simulink model "Fault_analysis_of_3phase"  (R2020a)
settings: Solver=VariableStepAuto  StartTime=0.0  StopTime=0.6  RelTol=1e-3
libraries: powerlib x6, simulink_extras x3
settings Model: Creator=Reaga  LastModifiedBy=Reaga
settings DebuggingCC: UnconnectedInputMsg=none  UnconnectedOutputMsg=none  UnconnectedLineMsg=none
settings ModelReferenceCC: EnableRefExpFcnMdlSchedulingChecks=off
settings RTWCC: Description=Generic Real-Time Target
settings ConfigComp: CovBoundaryAbsTol=1.0e-5

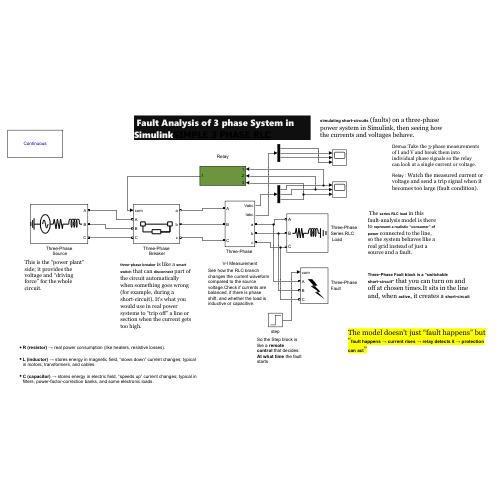
[thumbnail: Simulink's stored preview of the top-level diagram]
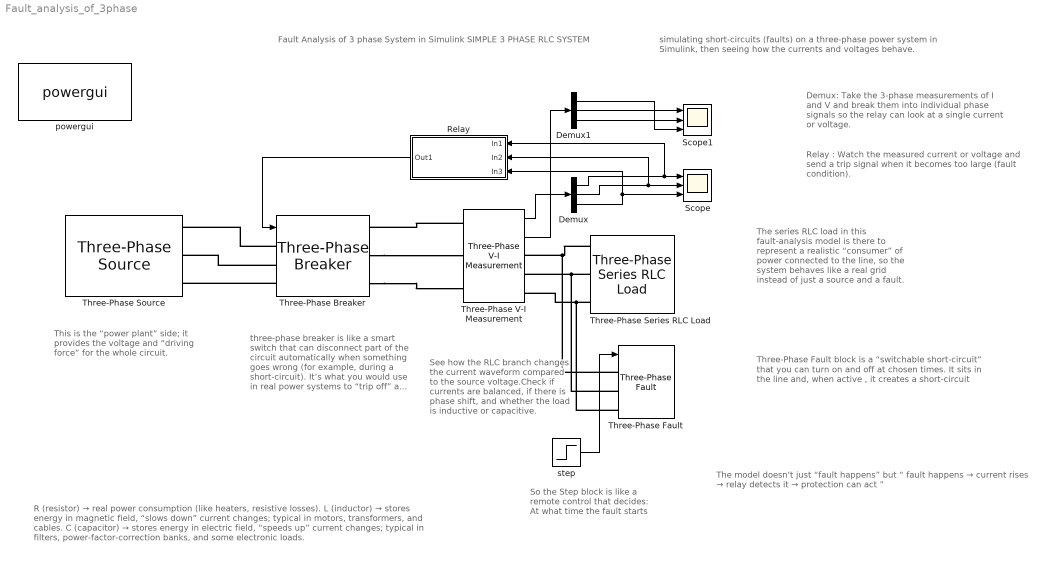
== system Fault_analysis_of_3phase ==
  note: The model doesn't just “fault happens” but “ fault happens → current rises → relay detects it → protection can act ”
  note: Relay : Watch the measured current or voltage and send a trip signal when it becomes too large (fault condition).
  note: Demux: Take the 3‑phase measurements of I and V and break them into individual phase signals so the relay can look at a single current or voltage.
  note: Three‑Phase Fault block is a “switchable short‑circuit” that you can turn on and off at chosen times. It sits in the line and, when active , it creates a short‑circuit
  note: So the Step block is like a remote control that decides:
      | At what time the fault starts
  note: The series RLC load in this fault‑analysis model is there to represent a realistic “consumer” of power connected to the line, so the system behaves like a real grid instead of just a source and a fault.
  note: three‑phase breaker is like a smart switch that can disconnect part of the circuit automatically when something goes wrong (for example, during a short‑circuit). It’s what you would use in real power systems to “trip off” a line or section when the current gets too high.
  note: simulating short‑circuits (faults) on a three‑phase power system in Simulink, then seeing how the currents and voltages behave.
  note: See how the RLC branch changes the current waveform compared to the source voltage.Check if currents are balanced, if there is phase shift, and whether the load is inductive or capacitive.
  note: R (resistor) → real power consumption (like heaters, resistive losses).
      | L (inductor) → stores energy in magnetic field, “slows down” current changes; typical in motors, transformers, and cables.
      | C (capacitor) → stores energy in electric field, “speeds up” current changes; typical in filters, power‑factor‑correction banks, and some electronic loads.
  note: This is the “power plant” side; it provides the voltage and “driving force” for the whole circuit.
  note: Fault Analysis of 3 phase System in Simulink SIMPLE 3 PHASE RLC SYSTEM
  Demux : Demux  Outputs=3
  Demux1 : Demux  Outputs=3
  "Relay " : Subsystem
  Scope : Scope  NumInputPorts=3
  Scope1 : Scope  NumInputPorts=3
  Three-Phase Breaker : powerlib/Elements/Three-Phase Breaker  InitialState=closed  SwitchA=on  SwitchB=on  SwitchC=on  SwitchTimes="[1/60  5/60]"  External=on  BreakerResistance=0.001  SnubberResistance=1e6  SnubberCapacitance=inf  Measurements=None
  Three-Phase Source : powerlib/Electrical Sources/Three-Phase Source  InternalConnection=Yg  VoltagePhases=off  Voltage=11e3  PhaseAngle=0  Voltage_phases=[25e3 25e3 25e3]/sqrt(3)  PhaseAngles_phases=[0 -120 +120]  Frequency=60  NonIdealSource=on  SpecifyImpedance=off  Resistance=1e-3  Inductance=1e-6  ShortCircuitLevel=100e6  BaseVoltage=11e3  XRratio=7  BusType=swing  Pref=10e3  Qref=0  Prefabc=[10e3, 10e3, 10e3]  Qrefabc=[0, 0, 0]  Qmin=-inf  Qmax=inf
  Three-Phase Series RLC Load : powerlib/Elements/Three-Phase Series RLC Load  LConnTagsString=A|B|C  Configuration=Y (grounded)  NominalVoltage=11e3  Vabc=[1e3 1e3 1e3]  Vabcp=[1e3 1e3 1e3]  NominalFrequency=50  UnbalancedPower=off  ActivePower=200e6  InductivePower=100  CapacitivePower=0  Pabc=[10e3 9e3 11e3]  QLabc=[100 90 110]  QCabc=[100 90 110]  Pabcp=[10e3 9e3 11e3]  QLabcp=[100 90 110]  QCabcp=[100 90 110]  Measurements=None  LoadType=constant Z
  Three-Phase V-I Measurement : powerlib/Measurements/Three-Phase V-I Measurement  VoltageMeasurement=phase-to-phase  SetLabelV=off  LabelV=Vabc  Vpu=off  VpuLL=off  CurrentMeasurement=yes  SetLabelI=off  LabelI=Iabc  Ipu=off  Pbase=100e6  Vbase=500e3  OutputType=Complex  PhasorSimulation=off  PSBequivalent=0
  Three-Phase Fault : powerlib/Elements/Three-Phase Fault  InitialStates=[0 0 0]  FaultA=on  FaultB=on  FaultC=on  GroundFault=on  SwitchTimes="[1/60  5/60]"  External=on  SwitchStatus=NaN  FaultResistance=0.001  GroundResistance=0.01  SnubberResistance=1e6  SnubberCapacitance=inf  Measurements=None
  powergui : powerlib/powergui  Priority=1  SimulationMode=Continuous  SampleTime=50e-6  frequency=60  Iterations=50  frequencyindice=60  Pbase=100e6  ErrMax=1e-4  UnitsV=kV  UnitsW=MW  buscounter=0  FunctionMessages=off  echomessages=off  EnableUseOfTLC=off  CurrentSourceSwitches=off  DisableSnubberDevices=off  DisableRonSwitches=off  DisableVfSwitches=off  DisplayEquations=off  AutomaticDiscreteSolvers=off  SolverType=Tustin/Backward Euler (TBE)  Interpol=off  ExternalGateDelay=off  methode=off  Ts=100  x0status=blocks  SPID=on  SwTol=0  HookPort=off  NonlinearTolerance=1e-4  nMaxIteration=100  ContinueOnMaxIteration=off  RestoreLinks=warning  ResistiveCurrentMeasurement=off  Frange=[0:2:500]  Ylog=off  Xlog=on  ShowGrid=off  save=off  variable=ZData  structure=0  ZoomFFT=off  StartTime=0.0  cycles=1  DisplayStyle=1  fundamental=60  FreqAxis=off  MaxFrequency=1000  frequencyindicesteady=1  RmsSteady=1  display=off
  step : Step  Time=0.1  SampleTime=0
  wires:
  step/1 -> Three-Phase Fault/1
  "Relay "/1(Out1) -> Three-Phase Breaker/1
  Demux1/1 -> Scope1/3
  Demux1/2 -> Scope1/1
  Demux1/3 -> Scope1/2
  Demux/1 -> "Relay "/1(In1), Scope/1
  Demux/2 -> "Relay "/2(In2), Scope/2
  Demux/3 -> "Relay "/3(In3), Scope/3
  Three-Phase V-I Measurement/1 -> Demux/1
  Three-Phase V-I Measurement/2 -> Demux1/1
  connections:
  Three-Phase Breaker/LConn1 -- Three-Phase Source/RConn1
  Three-Phase Breaker/LConn2 -- Three-Phase Source/RConn2
  Three-Phase Breaker/LConn3 -- Three-Phase Source/RConn3
  Three-Phase Series RLC Load/LConn2 -- Three-Phase Fault/LConn2 -- Three-Phase V-I Measurement/RConn2
  Three-Phase Series RLC Load/LConn1 -- Three-Phase Fault/LConn1 -- Three-Phase V-I Measurement/RConn1
  Three-Phase Series RLC Load/LConn3 -- Three-Phase Fault/LConn3 -- Three-Phase V-I Measurement/RConn3
  Three-Phase V-I Measurement/LConn1 -- Three-Phase Breaker/RConn1
  Three-Phase Breaker/RConn2 -- Three-Phase V-I Measurement/LConn2
  Three-Phase Breaker/RConn3 -- Three-Phase V-I Measurement/LConn3

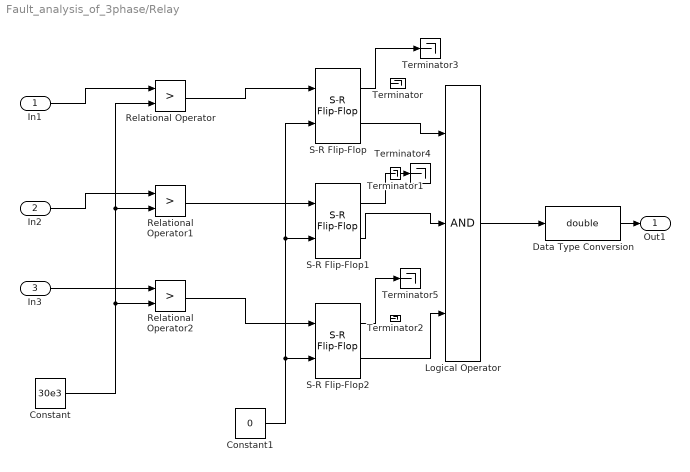
== system Fault_analysis_of_3phase/Relay  ==
  In1 : Inport
  In2 : Inport  Port=2
  In3 : Inport  Port=3
  Constant : Constant  Value=30e3
  Constant1 : Constant  Value=0  OutDataTypeStr=boolean
  Data Type Conversion : DataTypeConversion  OutDataTypeStr=double
  Logical Operator : Logic  Inputs=3  AllPortsSameDT=off  OutDataTypeStr=boolean
  Relational Operator : RelationalOperator  Operator=>  OutDataTypeStr=boolean  RndMeth=Nearest
  Relational Operator1 : RelationalOperator  Operator=>  OutDataTypeStr=boolean  RndMeth=Nearest
  Relational Operator2 : RelationalOperator  Operator=>  OutDataTypeStr=boolean  RndMeth=Nearest
  S-R Flip-Flop : simulink_extras/Flip Flops/S-R Flip-Flop  initial_condition=0
  S-R Flip-Flop1 : simulink_extras/Flip Flops/S-R Flip-Flop  initial_condition=0
  S-R Flip-Flop2 : simulink_extras/Flip Flops/S-R Flip-Flop  initial_condition=0
  Terminator{,1..5} (6 alike) : Terminator
  Out1 : Outport
  wires:
  In1/1 -> Relational Operator/1
  In2/1 -> Relational Operator1/1
  In3/1 -> Relational Operator2/1
  Constant/1 -> Relational Operator/2, Relational Operator1/2, Relational Operator2/2
  Relational Operator/1 -> S-R Flip-Flop/1
  Relational Operator1/1 -> S-R Flip-Flop1/1
  Relational Operator2/1 -> S-R Flip-Flop2/1
  Constant1/1 -> S-R Flip-Flop2/2, S-R Flip-Flop/2, S-R Flip-Flop1/2
  S-R Flip-Flop/2 -> Logical Operator/1
  S-R Flip-Flop1/2 -> Logical Operator/2
  S-R Flip-Flop2/2 -> Logical Operator/3
  S-R Flip-Flop2/1 -> Terminator5/1
  Logical Operator/1 -> Data Type Conversion/1
  Data Type Conversion/1 -> Out1/1
  S-R Flip-Flop/1 -> Terminator3/1
  S-R Flip-Flop1/1 -> Terminator4/1
